simulink library "PeripheralHandler"  (R2016b)
settings: Solver=VariableStepAuto  StartTime=0.0  StopTime=10.0  RelTol=1e-3
undefined symbols (not defined in the file or in its folder): ExoskeletonState, PDBCommand, waitTimeSitDown, waitTimeSlopeDown, waitTimeStairsDown, waitTimeStairsUp, waitTimeStandUp
libraries: simulink x1, ShutdownHandler x1
settings Model: Creator=march  LastModifiedBy=MARCH

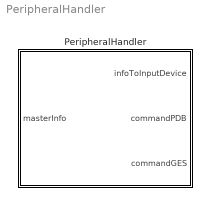
== system PeripheralHandler ==
  PeripheralHandler : Subsystem

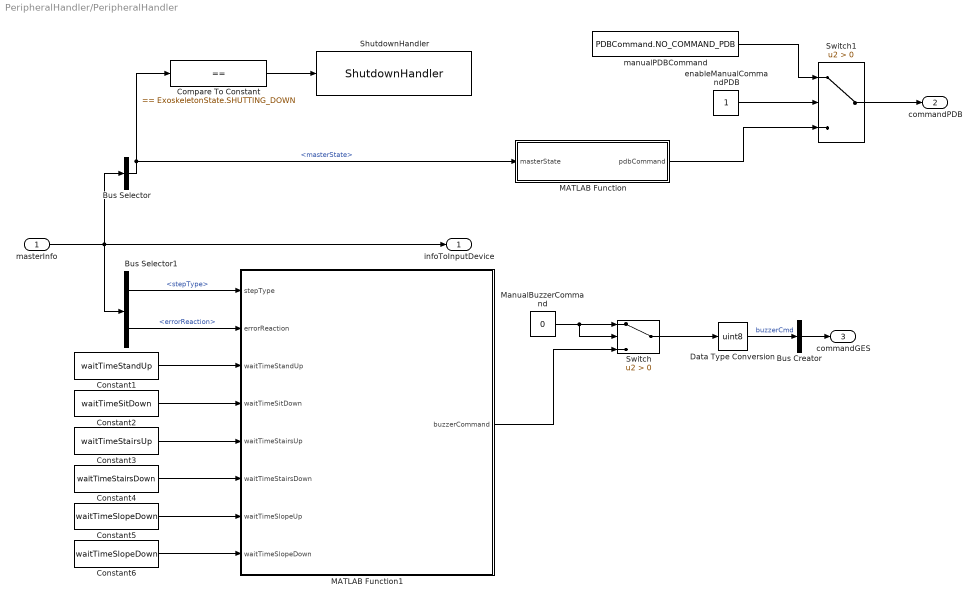
== system PeripheralHandler/PeripheralHandler ==
  masterInfo : Inport  OutDataTypeStr=Bus: MasterInfo
  Bus Creator : BusCreator  Inputs=1  OutDataTypeStr=Bus: GESCommand
  Bus Selector : BusSelector  OutputSignals=masterState
  Bus Selector1 : BusSelector  OutputSignals=stepType,errorReaction
  Compare To Constant : simulink/Logic and Bit Operations/Compare To Constant  relop===  const=ExoskeletonState.SHUTTING_DOWN  OutDataTypeStr=boolean
  Constant1 : Constant  Value=waitTimeStandUp  OutDataTypeStr=uint8
  Constant2 : Constant  Value=waitTimeSitDown  OutDataTypeStr=uint8
  Constant3 : Constant  Value=waitTimeStairsUp  OutDataTypeStr=uint8
  Constant4 : Constant  Value=waitTimeStairsDown  OutDataTypeStr=uint8
  Constant5 : Constant  Value=waitTimeSlopeDown  OutDataTypeStr=uint8
  Constant6 : Constant  Value=waitTimeSlopeDown  OutDataTypeStr=uint8
  Data Type Conversion : DataTypeConversion  OutDataTypeStr=uint8
  MATLAB Function : MATLAB Function  TreatAsAtomicUnit=on
  MATLAB Function1 : MATLAB Function  TreatAsAtomicUnit=on
  ManualBuzzerCommand : Constant  Value=0
  ShutdownHandler : ShutdownHandler/ShutdownHandler
  Switch : Switch  Criteria=u2 > Threshold
  Switch1 : Switch  Criteria=u2 > Threshold
  enableManualCommandPDB : Constant
  manualPDBCommand : Constant  Value=PDBCommand.NO_COMMAND_PDB
  infoToInputDevice : Outport
  commandPDB : Outport  Port=2
  commandGES : Outport  Port=3  OutDataTypeStr=Bus: GESCommand
  wires:
  manualPDBCommand/1 -> Switch1/1
  MATLAB Function/1(pdbCommand) -> Switch1/3
  Switch1/1 -> commandPDB/1
  enableManualCommandPDB/1 -> Switch1/2
  Bus Selector1/2 -> MATLAB Function1/2(errorReaction)  "<errorReaction>"
  Bus Selector1/1 -> MATLAB Function1/1(stepType)  "<stepType>"
  MATLAB Function1/1(buzzerCommand) -> Switch/3
  Switch/1 -> Data Type Conversion/1
  ManualBuzzerCommand/1 -> Switch/1, Switch/2
  Data Type Conversion/1 -> Bus Creator/1  "buzzerCmd"
  Bus Creator/1 -> commandGES/1
  Constant1/1 -> MATLAB Function1/3(waitTimeStandUp)
  Compare To Constant/1 -> ShutdownHandler/1
  Bus Selector/1 -> MATLAB Function/1(masterState), Compare To Constant/1  "<masterState>"
  masterInfo/1 -> infoToInputDevice/1, Bus Selector1/1, Bus Selector/1
  Constant2/1 -> MATLAB Function1/4(waitTimeSitDown)
  Constant3/1 -> MATLAB Function1/5(waitTimeStairsUp)
  Constant4/1 -> MATLAB Function1/6(waitTimeStairsDown)
  Constant6/1 -> MATLAB Function1/8(waitTimeSlopeDown)
  Constant5/1 -> MATLAB Function1/7(waitTimeSlopeUp)

== matlab function PeripheralHandler/MATLAB Function ==
  data: masterState input; pdbCommand output
function pdbCommand = getPDBCommandFromState(masterState)
% wrapper for getPDBCommandFromState
pdbCommand = getPDBCommandFromState(masterState);
end

== matlab function PeripheralHandler/MATLAB Function1 ==
  data: stepType input; errorReaction input; buzzerCommand output; waitTimeStandUp input; waitTimeSitDown input; waitTimeStairsUp input; waitTimeStairsDown input; waitTimeSlopeUp input; waitTimeSlopeDown input
function buzzerCommand = getBuzzerCommandFromState(stepType, errorReaction, waitTimeStandUp, waitTimeSitDown, waitTimeStairsUp, waitTimeStairsDown, waitTimeSlopeUp, waitTimeSlopeDown)
%Wrapper for getting buz command from master state 
buzzerCommand = getBuzzerCommandFromState(stepType, waitTimeStandUp, waitTimeSitDown, waitTimeStairsUp, waitTimeStairsDown, waitTimeSlopeUp, waitTimeSlopeDown, errorReaction);
end
